simulink model "gm_hdl_model_fixed_vnl"  (R2024a)
settings: Solver=FixedStepDiscrete  StartTime=0.0  StopTime=SIM_TIME  RelTol=1e-3
model workspace (MAT data in the model file):
  HDLVAXIManagerConfig : hdlverifier.internal.AXIMaster.ConfigParams (value not decoded)
undefined symbols (not defined in the file or in its folder): a, b, BUFFER_LEN, c, SAMPLING_FREQ, signal_1
libraries: hdlsllib x40, simulink x16, simulink_extras x5, dsphdlxfrm2 x2, dspsrcs4 x1
(part 3 of 3)

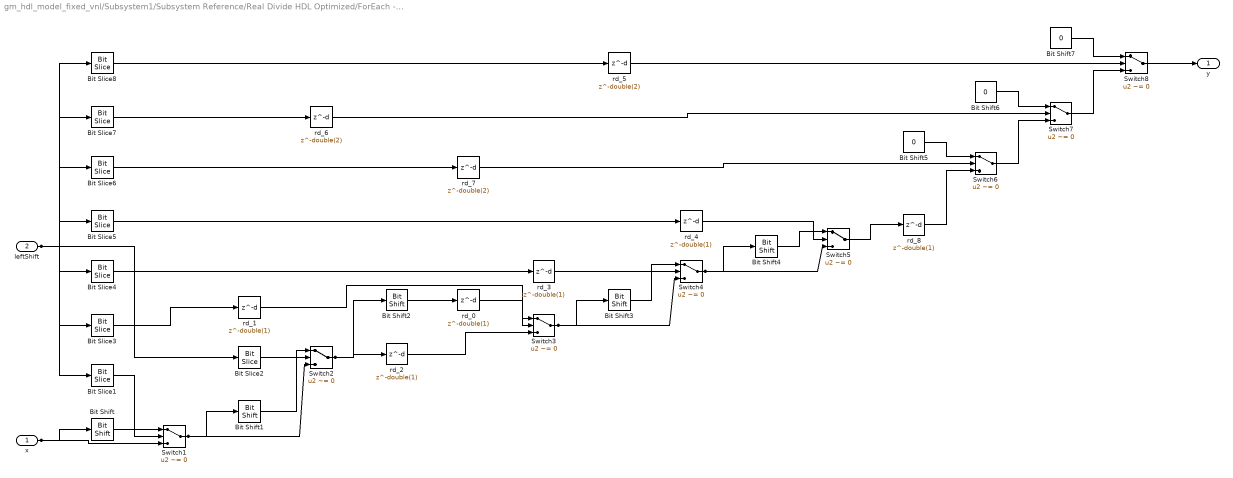
== system gm_hdl_model_fixed_vnl/Subsystem1/Subsystem Reference/Real Divide HDL Optimized/ForEach - Real Divide_instance1/Shift and cast to output type/Variable Left Shift ==
  x : Inport  OutDataTypeStr=fixdt(1, 23, 15)  SampleTime=1e-08
  leftShift : Inport  Port=2  OutDataTypeStr=int32  SampleTime=1e-08
  Bit Shift : hdlsllib/Logic and Bit Operations/Bit Shift  mode=Shift Left Logical  N=double(1)
  Bit Shift1 : hdlsllib/Logic and Bit Operations/Bit Shift  mode=Shift Left Logical  N=double(2)
  Bit Shift2 : hdlsllib/Logic and Bit Operations/Bit Shift  mode=Shift Left Logical  N=double(4)
  Bit Shift3 : hdlsllib/Logic and Bit Operations/Bit Shift  mode=Shift Left Logical  N=double(8)
  Bit Shift4 : hdlsllib/Logic and Bit Operations/Bit Shift  mode=Shift Left Logical  N=double(16)
  Bit Shift5 : Constant  Value=0  OutDataTypeStr=fixdt(1, 23, 15)  SampleTime=1e-08
  Bit Shift6 : Constant  Value=0  OutDataTypeStr=fixdt(1, 23, 15)  SampleTime=1e-08
  Bit Shift7 : Constant  Value=0  OutDataTypeStr=fixdt(1, 23, 15)  SampleTime=1e-08
  Bit Slice1 : hdlsllib/Logic and Bit Operations/Bit Slice  lidx=double(0)  ridx=double(0)
  Bit Slice2 : hdlsllib/Logic and Bit Operations/Bit Slice  lidx=double(1)  ridx=double(1)
  Bit Slice3 : hdlsllib/Logic and Bit Operations/Bit Slice  lidx=double(2)  ridx=double(2)
  Bit Slice4 : hdlsllib/Logic and Bit Operations/Bit Slice  lidx=double(3)  ridx=double(3)
  Bit Slice5 : hdlsllib/Logic and Bit Operations/Bit Slice  lidx=double(4)  ridx=double(4)
  Bit Slice6 : hdlsllib/Logic and Bit Operations/Bit Slice  lidx=double(5)  ridx=double(5)
  Bit Slice7 : hdlsllib/Logic and Bit Operations/Bit Slice  lidx=double(6)  ridx=double(6)
  Bit Slice8 : hdlsllib/Logic and Bit Operations/Bit Slice  lidx=double(7)  ridx=double(7)
  Switch{1..8} (8 alike) : Switch  Criteria=u2 ~= 0  Threshold=double(0)  OutDataTypeStr=fixdt(1, 23, 15)  SampleTime=1e-08  SaturateOnIntegerOverflow=off  InputSameDT=off
  rd_{0..4,8} (6 alike) : Delay  DelayLength=double(1)  InitialCondition=0  SampleTime=1e-08
  rd_5 : Delay  DelayLength=double(2)  InitialCondition=0  SampleTime=1e-08
  rd_6 : Delay  DelayLength=double(2)  InitialCondition=0  SampleTime=1e-08
  rd_7 : Delay  DelayLength=double(2)  InitialCondition=0  SampleTime=1e-08
  y : Outport  SampleTime=1e-08
  wires:
  rd_0/1 -> Switch3/1
  rd_1/1 -> Switch3/2
  rd_3/1 -> Switch4/2
  rd_4/1 -> Switch5/2
  rd_7/1 -> Switch6/2
  rd_6/1 -> Switch7/2
  rd_5/1 -> Switch8/2
  rd_2/1 -> Switch3/3
  rd_8/1 -> Switch6/3
  leftShift/1 -> Bit Slice8/1, Bit Slice7/1, Bit Slice6/1, Bit Slice5/1, Bit Slice4/1, Bit Slice3/1, Bit Slice2/1, Bit Slice1/1
  x/1 -> Switch1/3, Bit Shift/1
  Bit Shift/1 -> Switch1/1
  Bit Shift1/1 -> Switch2/1
  Bit Shift2/1 -> rd_0/1
  Bit Shift3/1 -> Switch4/1
  Bit Shift4/1 -> Switch5/1
  Bit Shift5/1 -> Switch6/1
  Bit Shift6/1 -> Switch7/1
  Bit Shift7/1 -> Switch8/1
  Bit Slice1/1 -> Switch1/2
  Bit Slice2/1 -> Switch2/2
  Bit Slice3/1 -> rd_1/1
  Bit Slice4/1 -> rd_3/1
  Bit Slice5/1 -> rd_4/1
  Bit Slice6/1 -> rd_7/1
  Bit Slice7/1 -> rd_6/1
  Bit Slice8/1 -> rd_5/1
  Switch1/1 -> Switch2/3, Bit Shift1/1
  Switch2/1 -> Bit Shift2/1, rd_2/1
  Switch3/1 -> Switch4/3, Bit Shift3/1
  Switch4/1 -> Switch5/3, Bit Shift4/1
  Switch5/1 -> rd_8/1
  Switch6/1 -> Switch7/3
  Switch7/1 -> Switch8/3
  Switch8/1 -> y/1

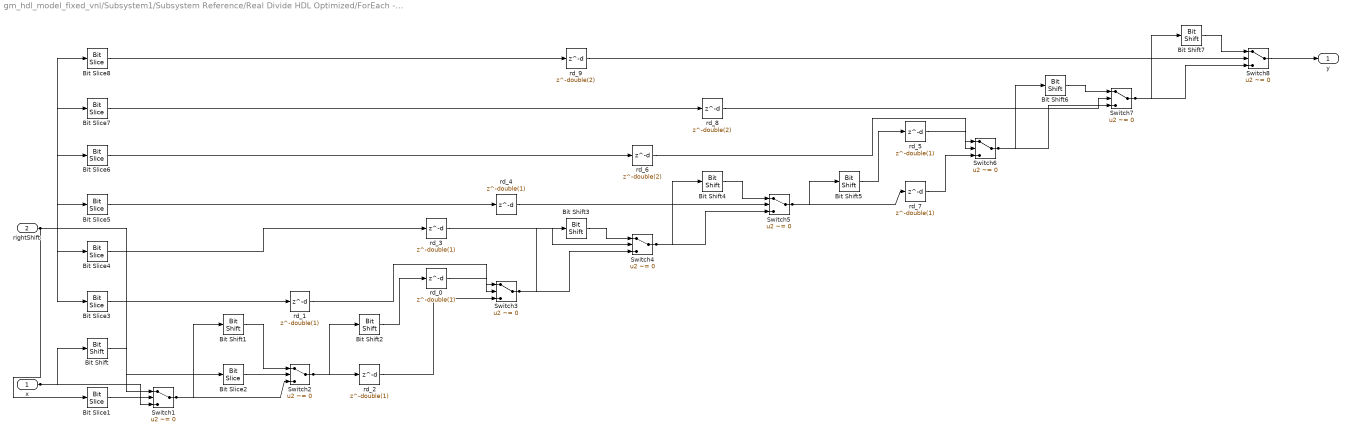
== system gm_hdl_model_fixed_vnl/Subsystem1/Subsystem Reference/Real Divide HDL Optimized/ForEach - Real Divide_instance1/Shift and cast to output type/Variable Right Shift ==
  x : Inport  OutDataTypeStr=fixdt(1, 23, 15)  SampleTime=1e-08
  rightShift : Inport  Port=2  OutDataTypeStr=int32  SampleTime=1e-08
  Bit Shift : hdlsllib/Logic and Bit Operations/Bit Shift  mode=Shift Right Arithmetic  N=double(1)
  Bit Shift1 : hdlsllib/Logic and Bit Operations/Bit Shift  mode=Shift Right Arithmetic  N=double(2)
  Bit Shift2 : hdlsllib/Logic and Bit Operations/Bit Shift  mode=Shift Right Arithmetic  N=double(4)
  Bit Shift3 : hdlsllib/Logic and Bit Operations/Bit Shift  mode=Shift Right Arithmetic  N=double(8)
  Bit Shift4 : hdlsllib/Logic and Bit Operations/Bit Shift  mode=Shift Right Arithmetic  N=double(16)
  Bit Shift5 : hdlsllib/Logic and Bit Operations/Bit Shift  mode=Shift Right Arithmetic  N=double(22)
  Bit Shift6 : hdlsllib/Logic and Bit Operations/Bit Shift  mode=Shift Right Arithmetic  N=double(22)
  Bit Shift7 : hdlsllib/Logic and Bit Operations/Bit Shift  mode=Shift Right Arithmetic  N=double(22)
  Bit Slice1 : hdlsllib/Logic and Bit Operations/Bit Slice  lidx=double(0)  ridx=double(0)
  Bit Slice2 : hdlsllib/Logic and Bit Operations/Bit Slice  lidx=double(1)  ridx=double(1)
  Bit Slice3 : hdlsllib/Logic and Bit Operations/Bit Slice  lidx=double(2)  ridx=double(2)
  Bit Slice4 : hdlsllib/Logic and Bit Operations/Bit Slice  lidx=double(3)  ridx=double(3)
  Bit Slice5 : hdlsllib/Logic and Bit Operations/Bit Slice  lidx=double(4)  ridx=double(4)
  Bit Slice6 : hdlsllib/Logic and Bit Operations/Bit Slice  lidx=double(5)  ridx=double(5)
  Bit Slice7 : hdlsllib/Logic and Bit Operations/Bit Slice  lidx=double(6)  ridx=double(6)
  Bit Slice8 : hdlsllib/Logic and Bit Operations/Bit Slice  lidx=double(7)  ridx=double(7)
  Switch{1..8} (8 alike) : Switch  Criteria=u2 ~= 0  Threshold=double(0)  OutDataTypeStr=fixdt(1, 23, 15)  SampleTime=1e-08  SaturateOnIntegerOverflow=off  InputSameDT=off
  rd_{0..5,7} (7 alike) : Delay  DelayLength=double(1)  InitialCondition=0  SampleTime=1e-08
  rd_6 : Delay  DelayLength=double(2)  InitialCondition=0  SampleTime=1e-08
  rd_8 : Delay  DelayLength=double(2)  InitialCondition=0  SampleTime=1e-08
  rd_9 : Delay  DelayLength=double(2)  InitialCondition=0  SampleTime=1e-08
  y : Outport  SampleTime=1e-08
  wires:
  rd_0/1 -> Switch3/1
  rd_5/1 -> Switch6/1
  rd_1/1 -> Switch3/2
  rd_3/1 -> Switch4/2
  rd_4/1 -> Switch5/2
  rd_6/1 -> Switch6/2
  rd_8/1 -> Switch7/2
  rd_9/1 -> Switch8/2
  rd_2/1 -> Switch3/3
  rd_7/1 -> Switch6/3
  rightShift/1 -> Bit Slice8/1, Bit Slice7/1, Bit Slice6/1, Bit Slice5/1, Bit Slice4/1, Bit Slice3/1, Bit Slice2/1, Bit Slice1/1
  x/1 -> Switch1/3, Bit Shift/1
  Bit Shift/1 -> Switch1/1
  Bit Shift1/1 -> Switch2/1
  Bit Shift2/1 -> rd_0/1
  Bit Shift3/1 -> Switch4/1
  Bit Shift4/1 -> Switch5/1
  Bit Shift5/1 -> rd_5/1
  Bit Shift6/1 -> Switch7/1
  Bit Shift7/1 -> Switch8/1
  Bit Slice1/1 -> Switch1/2
  Bit Slice2/1 -> Switch2/2
  Bit Slice3/1 -> rd_1/1
  Bit Slice4/1 -> rd_3/1
  Bit Slice5/1 -> rd_4/1
  Bit Slice6/1 -> rd_6/1
  Bit Slice7/1 -> rd_8/1
  Bit Slice8/1 -> rd_9/1
  Switch1/1 -> Switch2/3, Bit Shift1/1
  Switch2/1 -> Bit Shift2/1, rd_2/1
  Switch3/1 -> Switch4/3, Bit Shift3/1
  Switch4/1 -> Switch5/3, Bit Shift4/1
  Switch5/1 -> Bit Shift5/1, rd_7/1
  Switch6/1 -> Switch7/3, Bit Shift6/1
  Switch7/1 -> Switch8/3, Bit Shift7/1
  Switch8/1 -> y/1

== system gm_hdl_model_fixed_vnl/Subsystem1/myRMS/CORDIC Square Root HDL Optimized/Synchronous Subsystem/cordicSquareRootHDL/embmathops_c2_s84XJG1CWMolALoedlonStG_cordicSquareRootHDL_controlled ==
  in0 : Inport  OutDataTypeStr=fixdt(0, 16, 7)  SampleTime=1e-08
  in1 : Inport  Port=2  OutDataTypeStr=boolean  SampleTime=1e-08
  in2 : Inport  Port=3  OutDataTypeStr=boolean  SampleTime=1e-08
  stateControl : EnablePort  OutDataTypeStr=boolean
  embmathops_c2_s84XJG1CWMolALoedlonStG_cordicSquareRootHDL : MATLAB Function  TreatAsAtomicUnit=on
      settings: LibrarySourceBlock=embmathops/CORDIC Square Root HDL Optimized/Synchronous Subsystem/cordicSquareRootHDL
  out0 : Outport  OutDataTypeStr=fixdt(1, 16, 14)  SampleTime=1e-08  InitialOutput=0
  out1 : Outport  Port=2  OutDataTypeStr=int32  SampleTime=1e-08  InitialOutput=0
  out2 : Outport  Port=3  OutDataTypeStr=boolean  SampleTime=1e-08  InitialOutput=0
  out3 : Outport  Port=4  OutDataTypeStr=boolean  SampleTime=1e-08  InitialOutput=0
  wires:
  in2/1 -> embmathops_c2_s84XJG1CWMolALoedlonStG_cordicSquareRootHDL/3(restart)
  in1/1 -> embmathops_c2_s84XJG1CWMolALoedlonStG_cordicSquareRootHDL/2(validIn)
  in0/1 -> embmathops_c2_s84XJG1CWMolALoedlonStG_cordicSquareRootHDL/1(u)
  embmathops_c2_s84XJG1CWMolALoedlonStG_cordicSquareRootHDL/4(validOut) -> out3/1
  embmathops_c2_s84XJG1CWMolALoedlonStG_cordicSquareRootHDL/3(isZero) -> out2/1
  embmathops_c2_s84XJG1CWMolALoedlonStG_cordicSquareRootHDL/2(eOut) -> out1/1
  embmathops_c2_s84XJG1CWMolALoedlonStG_cordicSquareRootHDL/1(dataOut) -> out0/1

== system gm_hdl_model_fixed_vnl/Subsystem1/Subsystem Reference/Absolute of Complex/CORDIC Square Root HDL Optimized1/Synchronous Subsystem/cordicSquareRootHDL/embmathops_c2_srwrzER3uCGRdPfDbow0ID_cordicSquareRootHDL_controlled ==
  in0 : Inport  OutDataTypeStr=fixdt(1, 24, 22)  SampleTime=1e-08
  in1 : Inport  Port=2  OutDataTypeStr=boolean  SampleTime=1e-08
  in2 : Inport  Port=3  OutDataTypeStr=boolean  SampleTime=1e-08
  stateControl : EnablePort  OutDataTypeStr=boolean
  embmathops_c2_srwrzER3uCGRdPfDbow0ID_cordicSquareRootHDL : MATLAB Function  TreatAsAtomicUnit=on
      settings: LibrarySourceBlock=embmathops/CORDIC Square Root HDL Optimized/Synchronous Subsystem/cordicSquareRootHDL
  out0 : Outport  OutDataTypeStr=fixdt(1, 24, 22)  SampleTime=1e-08  InitialOutput=0
  out1 : Outport  Port=2  OutDataTypeStr=int32  SampleTime=1e-08  InitialOutput=0
  out2 : Outport  Port=3  OutDataTypeStr=boolean  SampleTime=1e-08  InitialOutput=0
  out3 : Outport  Port=4  OutDataTypeStr=boolean  SampleTime=1e-08  InitialOutput=0
  wires:
  in2/1 -> embmathops_c2_srwrzER3uCGRdPfDbow0ID_cordicSquareRootHDL/3(restart)
  in1/1 -> embmathops_c2_srwrzER3uCGRdPfDbow0ID_cordicSquareRootHDL/2(validIn)
  in0/1 -> embmathops_c2_srwrzER3uCGRdPfDbow0ID_cordicSquareRootHDL/1(u)
  embmathops_c2_srwrzER3uCGRdPfDbow0ID_cordicSquareRootHDL/4(validOut) -> out3/1
  embmathops_c2_srwrzER3uCGRdPfDbow0ID_cordicSquareRootHDL/3(isZero) -> out2/1
  embmathops_c2_srwrzER3uCGRdPfDbow0ID_cordicSquareRootHDL/2(eOut) -> out1/1
  embmathops_c2_srwrzER3uCGRdPfDbow0ID_cordicSquareRootHDL/1(dataOut) -> out0/1

== system gm_hdl_model_fixed_vnl/Subsystem1/Subsystem Reference/Real Divide HDL Optimized/ForEach - Real Divide_instance1/Divide real numerator by denominator/normalizedCORDICDivide/embreciprocals_c21_normalizedCORDICDivide_controlled ==
  in0 : Inport  OutDataTypeStr=fixdt(1, 17, 15)  SampleTime=1e-08
  in1 : Inport  Port=2  OutDataTypeStr=fixdt(1, 17, 15)  SampleTime=1e-08
  in2 : Inport  Port=3  OutDataTypeStr=fixdt(1, 33, 0)  SampleTime=1e-08
  in3 : Inport  Port=4  OutDataTypeStr=int32  SampleTime=1e-08
  in4 : Inport  Port=5  OutDataTypeStr=boolean  SampleTime=1e-08
  in5 : Inport  Port=6  OutDataTypeStr=boolean  SampleTime=1e-08
  in6 : Inport  Port=7  OutDataTypeStr=boolean  SampleTime=1e-08
  stateControl : EnablePort  OutDataTypeStr=boolean
  embreciprocals_c21_normalizedCORDICDivide : MATLAB Function  TreatAsAtomicUnit=on
      settings: LibrarySourceBlock=embreciprocals/Divide real numerator by denominator/normalizedCORDICDivide
  out0 : Outport  OutDataTypeStr=fixdt(1, 17, 15)  SampleTime=1e-08  InitialOutput=0
  out1 : Outport  Port=2  OutDataTypeStr=fixdt(1, 34, 0)  SampleTime=1e-08  InitialOutput=0
  out2 : Outport  Port=3  OutDataTypeStr=boolean  SampleTime=1e-08  InitialOutput=0
  out3 : Outport  Port=4  OutDataTypeStr=boolean  SampleTime=1e-08  InitialOutput=0
  wires:
  in6/1 -> embreciprocals_c21_normalizedCORDICDivide/7(validIn)
  in5/1 -> embreciprocals_c21_normalizedCORDICDivide/6(isDenNegative)
  in4/1 -> embreciprocals_c21_normalizedCORDICDivide/5(isNumNegative)
  in3/1 -> embreciprocals_c21_normalizedCORDICDivide/4(tDen)
  in2/1 -> embreciprocals_c21_normalizedCORDICDivide/3(tNum)
  in1/1 -> embreciprocals_c21_normalizedCORDICDivide/2(den)
  in0/1 -> embreciprocals_c21_normalizedCORDICDivide/1(num)
  embreciprocals_c21_normalizedCORDICDivide/4(validOut) -> out3/1
  embreciprocals_c21_normalizedCORDICDivide/3(isDenZeroOut) -> out2/1
  embreciprocals_c21_normalizedCORDICDivide/2(t) -> out1/1
  embreciprocals_c21_normalizedCORDICDivide/1(y) -> out0/1

== system gm_hdl_model_fixed_vnl/Subsystem1/Subsystem Reference/Real Divide HDL Optimized/ForEach - Real Divide_instance1/Normalize denominator/positiveRealNormalizer/embreciprocals_c3_positiveRealNormalizer_controlled ==
  in0 : Inport  OutDataTypeStr=fixdt(1, 17, 14)  SampleTime=1e-08
  in1 : Inport  Port=2  OutDataTypeStr=boolean  SampleTime=1e-08
  stateControl : EnablePort  OutDataTypeStr=boolean
  embreciprocals_c3_positiveRealNormalizer : MATLAB Function  TreatAsAtomicUnit=on
      settings: LibrarySourceBlock=embreciprocals/Real Normalizer HDL Optimized/positiveRealNormalizer
  out0 : Outport  OutDataTypeStr=fixdt(1, 17, 15)  SampleTime=1e-08  InitialOutput=0
  out1 : Outport  Port=2  OutDataTypeStr=int32  SampleTime=1e-08  InitialOutput=0
  out2 : Outport  Port=3  OutDataTypeStr=boolean  SampleTime=1e-08  InitialOutput=0
  out3 : Outport  Port=4  OutDataTypeStr=boolean  SampleTime=1e-08  InitialOutput=0
  wires:
  in1/1 -> embreciprocals_c3_positiveRealNormalizer/2(validIn)
  in0/1 -> embreciprocals_c3_positiveRealNormalizer/1(u)
  embreciprocals_c3_positiveRealNormalizer/4(validOut) -> out3/1
  embreciprocals_c3_positiveRealNormalizer/3(isNegative) -> out2/1
  embreciprocals_c3_positiveRealNormalizer/2(e) -> out1/1
  embreciprocals_c3_positiveRealNormalizer/1(x) -> out0/1

== system gm_hdl_model_fixed_vnl/Subsystem1/Subsystem Reference/Real Divide HDL Optimized/ForEach - Real Divide_instance1/Normalize numerator/positiveRealNormalizer/embreciprocals_c3_positiveRealNormalizer_controlled ==
  in0 : Inport  OutDataTypeStr=fixdt(1, 17, 14)  SampleTime=1e-08
  in1 : Inport  Port=2  OutDataTypeStr=boolean  SampleTime=1e-08
  stateControl : EnablePort  OutDataTypeStr=boolean
  embreciprocals_c3_positiveRealNormalizer : MATLAB Function  TreatAsAtomicUnit=on
      settings: LibrarySourceBlock=embreciprocals/Real Normalizer HDL Optimized/positiveRealNormalizer
  out0 : Outport  OutDataTypeStr=fixdt(1, 17, 15)  SampleTime=1e-08  InitialOutput=0
  out1 : Outport  Port=2  OutDataTypeStr=int32  SampleTime=1e-08  InitialOutput=0
  out2 : Outport  Port=3  OutDataTypeStr=boolean  SampleTime=1e-08  InitialOutput=0
  out3 : Outport  Port=4  OutDataTypeStr=boolean  SampleTime=1e-08  InitialOutput=0
  wires:
  in1/1 -> embreciprocals_c3_positiveRealNormalizer/2(validIn)
  in0/1 -> embreciprocals_c3_positiveRealNormalizer/1(u)
  embreciprocals_c3_positiveRealNormalizer/4(validOut) -> out3/1
  embreciprocals_c3_positiveRealNormalizer/3(isNegative) -> out2/1
  embreciprocals_c3_positiveRealNormalizer/2(e) -> out1/1
  embreciprocals_c3_positiveRealNormalizer/1(x) -> out0/1

== matlab function gm_hdl_model_fixed_vnl/Subsystem1/Subsystem Reference/Real Divide HDL Optimized/ForEach - Real Divide_instance1/Normalize numerator/positiveRealNormalizer/embreciprocals_c3_positiveRealNormalizer_controlled/embreciprocals_c3_positiveRealNormalizer ==
  settings: fimath=hdlfimath
  data: u input; x output; validIn input; e output; isNegative output; validOut output
function [x, e, isNegative, validOut] = realNormalizer(u, validIn)
    %realNormalizer Normalize real values.
    % Given real scalar u ~= 0, this block produces x such that
    %    1 <= x < 2,
    % e such that
    %    x = (2^e)*|u|,
    % and isNegative = u<0.
    %
    %   When u = 0 and u is fixed-point or scaled-double, then x = 0 and
    %   e = (2^nextpow2(x.WordLength)) - x.WordLength - x.FractionLength.
    %
    %   When u = 0 and u is floating-point, then x = 0 and e = 1.
    
    %   Copyright 2019 The MathWorks, Inc.
    %#codegen
    
    % This function only works on scalars.
    % Only operate on the real part
    fixed.internal.reciprocal.validateNormalizerInputs(u, validIn);
    % Normalize in unsigned type.
    [x_normalized, n_normalized, isNegative, validOut] = normalize(real(u), validIn);
    % Cast the output to signed if the input was signed.
    x = fixed.internal.reciprocal.castToInputSignedness(x_normalized,u);
    % Convert the normalized shift value based on the data type of the
    % input U so that the output of the normalizer X is in real-world
    % scale and X = (2^N)*U.
    e = fi(int32(0));
    e(:) = fixed.internal.reciprocal.normalizedShiftToRealWorldValueShift(n_normalized,u);
end

function [x_normalized, e_normalized, isNegative, validOut] = normalize(u, validIn)
    [u, isNegative] = fixed.reciprocal.pipelined.makeRealScalarPositive(u);
    if isfi(u) && isfixed(u)
        % Normalize fixed-point values
        [x_normalized, e_normalized, isNegative, validOut] = normalizeFixedpoint(u, isNegative, validIn);
    else
        % Normalize floating-point or scaled-double
        [x_normalized, e_normalized, validOut] = fixed.internal.reciprocal.normalizePositiveFloatOrScaledDouble(u, validIn);
    end
end

function [u_normalized, e_normalized, isNegativeOut, validOut] = normalizeFixedpoint(u, isNegative, validIn)
    % Normalize fixed-point values.
    persistent validReg
    persistent tReg
    persistent xReg
    persistent isNegativeReg
    % For fixed-point types, the normalization uses a binary search of
    % length log2 of the word length of the input.
    number_of_stages = coder.const(nextpow2(u.WordLength));
    
    if isempty(validReg)
        validReg = false(number_of_stages+1,1);
        tReg = zeros(number_of_stages+1,1,'like',fi(0,0,max(number_of_stages,1),0));
        xReg = zeros(number_of_stages+1,1,'like',fi([],0,u.WordLength,0));
        isNegativeReg = false(number_of_stages+1,1);
    end
    
    [u_normalized, e_normalized,validOut,...
        validReg, tReg,xReg...  % Persistent
        ] = fixed.internal.reciprocal.normalizePositiveFixedPoint(u, validIn, number_of_stages, ...
        validReg, tReg,xReg...  % Persistent
        );
    % Assign outputs from states
    isNegativeOut = isNegativeReg(end);
    
    % Update isNegative states
    coder.unroll;
    for k = number_of_stages:-1:1
        isNegativeReg(k+1) = isNegativeReg(k);
    end
    isNegativeReg(1) = isNegative;
end

== matlab function gm_hdl_model_fixed_vnl/Subsystem1/Subsystem Reference/Real Divide HDL Optimized/Reshape to original size/embreciprocals_c11_Reshape_to_original_size ==
  data: y input; u input; z output
function z = reshape_to_original_size(y,u)
    z = reshape(y,size(u));
end

== matlab function gm_hdl_model_fixed_vnl/Subsystem1/Subsystem Reference/Real Divide HDL Optimized/ForEach - Real Divide_instance1/Normalize denominator/positiveRealNormalizer/embreciprocals_c3_positiveRealNormalizer_controlled/embreciprocals_c3_positiveRealNormalizer ==
  settings: fimath=hdlfimath
  data: u input; x output; validIn input; e output; isNegative output; validOut output
function [x, e, isNegative, validOut] = realNormalizer(u, validIn)
    %realNormalizer Normalize real values.
    % Given real scalar u ~= 0, this block produces x such that
    %    1 <= x < 2,
    % e such that
    %    x = (2^e)*|u|,
    % and isNegative = u<0.
    %
    %   When u = 0 and u is fixed-point or scaled-double, then x = 0 and
    %   e = (2^nextpow2(x.WordLength)) - x.WordLength - x.FractionLength.
    %
    %   When u = 0 and u is floating-point, then x = 0 and e = 1.
    
    %   Copyright 2019 The MathWorks, Inc.
    %#codegen
    
    % This function only works on scalars.
    % Only operate on the real part
    fixed.internal.reciprocal.validateNormalizerInputs(u, validIn);
    % Normalize in unsigned type.
    [x_normalized, n_normalized, isNegative, validOut] = normalize(real(u), validIn);
    % Cast the output to signed if the input was signed.
    x = fixed.internal.reciprocal.castToInputSignedness(x_normalized,u);
    % Convert the normalized shift value based on the data type of the
    % input U so that the output of the normalizer X is in real-world
    % scale and X = (2^N)*U.
    e = fi(int32(0));
    e(:) = fixed.internal.reciprocal.normalizedShiftToRealWorldValueShift(n_normalized,u);
end

function [x_normalized, e_normalized, isNegative, validOut] = normalize(u, validIn)
    [u, isNegative] = fixed.reciprocal.pipelined.makeRealScalarPositive(u);
    if isfi(u) && isfixed(u)
        % Normalize fixed-point values
        [x_normalized, e_normalized, isNegative, validOut] = normalizeFixedpoint(u, isNegative, validIn);
    else
        % Normalize floating-point or scaled-double
        [x_normalized, e_normalized, validOut] = fixed.internal.reciprocal.normalizePositiveFloatOrScaledDouble(u, validIn);
    end
end

function [u_normalized, e_normalized, isNegativeOut, validOut] = normalizeFixedpoint(u, isNegative, validIn)
    % Normalize fixed-point values.
    persistent validReg
    persistent tReg
    persistent xReg
    persistent isNegativeReg
    % For fixed-point types, the normalization uses a binary search of
    % length log2 of the word length of the input.
    number_of_stages = coder.const(nextpow2(u.WordLength));
    
    if isempty(validReg)
        validReg = false(number_of_stages+1,1);
        tReg = zeros(number_of_stages+1,1,'like',fi(0,0,max(number_of_stages,1),0));
        xReg = zeros(number_of_stages+1,1,'like',fi([],0,u.WordLength,0));
        isNegativeReg = false(number_of_stages+1,1);
    end
    
    [u_normalized, e_normalized,validOut,...
        validReg, tReg,xReg...  % Persistent
        ] = fixed.internal.reciprocal.normalizePositiveFixedPoint(u, validIn, number_of_stages, ...
        validReg, tReg,xReg...  % Persistent
        );
    % Assign outputs from states
    isNegativeOut = isNegativeReg(end);
    
    % Update isNegative states
    coder.unroll;
    for k = number_of_stages:-1:1
        isNegativeReg(k+1) = isNegativeReg(k);
    end
    isNegativeReg(1) = isNegative;
end

== matlab function gm_hdl_model_fixed_vnl/Subsystem1/Subsystem Reference/Real Divide HDL Optimized/ForEach - Real Divide_instance1/Upcast Wordlength/slutils_c2_Upcast_Wordlength ==
  data: x input; u output; y input; v output
function [u, v] = upcastWordlength(x, y)

% Copyright 2019 The MathWorks, Inc.

%#codegen

[u, v] = fixed.internal.type.upcastWordlength(x,y);

end

== matlab function gm_hdl_model_fixed_vnl/Subsystem1/Subsystem Reference/Real Divide HDL Optimized/ForEach - Real Divide_instance1/MATLAB Function/embreciprocals_c13_MATLAB_Function ==
  settings: fimath=hdlfimath
  data: num input; num_out output; t_num input; t_num_out output
function [num_out, t_num_out] = fcn(num, t_num)

num_out = bitsra(num,1);
t_num_out = t_num - 1;

end

== matlab function gm_hdl_model_fixed_vnl/Subsystem1/myRMS/CORDIC Square Root HDL Optimized/Synchronous Subsystem/cordicSquareRootHDL/embmathops_c2_s84XJG1CWMolALoedlonStG_cordicSquareRootHDL_controlled/embmathops_c2_s84XJG1CWMolALoedlonStG_cordicSquareRootHDL ==
  settings: fimath=hdlfimath
  data: u input; dataOut output; validIn input; restart input; eOut output; isZero output; validOut output; maximumShiftValue parameter; nIterPerReg parameter; autoMaximumShiftVal parameter
function [dataOut,eOut,isZero,validOut] = cordicSquareRootHDL(u,validIn,restart,maximumShiftValue, nIterPerReg, autoMaximumShiftVal)
    % [dataOut,eOut,validOut] = cordicSquareRootHDL(u,validIn,restart,maximumShiftValue,nIterPerReg)
    % This function computes the normalized square root of input data u
    % based on CORDIC hyperbolic vectoring mode. eOut is the bit shift
    % value to be used during denormalization.
    %
    % This function first performs normalization of input u and then
    % computes square root of normalized u using CORDIC hyperbolic
    % vectoring mode.

    %   Copyright 2023 The MathWorks, Inc.

    %#codegen
    
    fixed.internal.reciprocal.validateNormalizerInputs(u, validIn);

    %% Constants
    if autoMaximumShiftVal
        N = coder.const(fixed.cordic.maximumShiftValue(u));
    else
        N = coder.const(maximumShiftValue);
    end

    Kn = coder.const(fixed.cordic.hyperbolic.inverseScaleFactor(N));
    INITOFFSET = coder.const(0.25);
    shiftSeq = coder.const(fixed.cordic.hyperbolic.shiftSequence(N));
    nCORDICIterations = coder.const(length(shiftSeq));

    %% Run CORDIC square root workflow
    uPos = fixed.cordic.linear.makeRealScalarPositiveUnsigned(u);
    if isfi(u)&&isscaledtype(u)
        coder.internal.assert(u.WordLength>N,'fixed:emblib:CORDICMaxShiftValMustBeSmallerThanWordlength');
        [dataOut, eOut, isZero, validOut] = sqrtIterFixed(uPos, validIn, restart,nIterPerReg,Kn,INITOFFSET,shiftSeq,nCORDICIterations);
    else
        [dataOut, eOut] = fixed.emblib.cordicsqrt.cordicSqrtFloat(uPos, Kn, INITOFFSET, shiftSeq, nCORDICIterations);
        validOut = validIn;
        isZero = u==0;
    end
end

function [dataOut, eOut, isZero, validOut] = sqrtIterFixed(u, validIn, restart, nIterPerReg, Kn, INITOFFSET, shiftSeq, nCORDICIterations)
        uInt = stripscaling(u);
        
        wordLength = coder.const(uInt.WordLength);
        normalizerType = numerictype(1,32,0);

        % CORDIC datatype and corresponding fimath
        CORDICprototype = fi([],1,wordLength,wordLength-2,'DataType',uInt.DataType);
        Fxy = fixed.fimathLike(CORDICprototype);
        
        % Allocate registers
        [numOfNormSteps,nNormReg,normInd,nTrailingNormSteps,trailingNormIdx,nLeadingCORDICSteps,nCORDICReg,CORDICShiftInd,nTotReg]...
            = fixed.emblib.cordicsqrt.allocateReg(wordLength,nCORDICIterations,nIterPerReg);
        
        %% Registers
        persistent xRegNorm xRegCORDIC yReg eRegNorm eRegCORDIC validReg dataOutReg eOutReg isZeroReg
        if isempty(xRegNorm)
            xRegNorm = zeros(nNormReg,1,'like',uInt);
            xRegCORDIC = setfimath(zeros(nCORDICReg,1,'like',CORDICprototype),Fxy);
            yReg = setfimath(zeros(nCORDICReg,1,'like',CORDICprototype),Fxy);
            eRegNorm = fi(zeros(nNormReg,1),0,numOfNormSteps,0);
            eRegCORDIC = fi(zeros(nCORDICReg,1),normalizerType);
            validReg = false(nTotReg+1,1);
            dataOutReg = setfimath(cast(0,'like',CORDICprototype),Fxy);
            eOutReg = fi(0,normalizerType);
            isZeroReg = false(nTotReg+1,1);
        end
        
        %% Assign outputs
        dataOut = dataOutReg;
        eOut = eOutReg;
        validOut = validReg(end);
        isZero = isZeroReg(end);
        
        %% Update registers
        [xRegNorm, xRegCORDIC, yReg, eRegNorm, eRegCORDIC, validReg, dataOutReg, eOutReg, isZeroReg]...
        = fixed.emblib.cordicsqrt.cordicSqrtFiScaledtypeUpdateReg(u, uInt, validIn, restart,... % Inputs
        xRegNorm, xRegCORDIC, yReg, eRegNorm, eRegCORDIC, validReg, dataOutReg, eOutReg, isZeroReg,... %Registers
        Kn, INITOFFSET, shiftSeq, nIterPerReg,... % Constants for algorithms
        nTotReg, nNormReg, CORDICShiftInd, normInd, nTrailingNormSteps, trailingNormIdx, nLeadingCORDICSteps); % Constants for partition algorithms
end

== matlab function gm_hdl_model_fixed_vnl/Subsystem1/BUF_MIN_MAX_AVG/MATLAB Function1/MATLAB Function1 ==
  data: input_data input; max_out output; reset input
function max_out = stream_max(input_data, reset)
    % input_data: Input data stream (e.g., 16-bit integer)
    % reset: Reset signal (active high)

    % Persistent variable to hold the current maximum value
    persistent current_max;
    
    % Initialize persistent variable if it's the first time the function is called
    if isempty(current_max)
        current_max = fi(-0.5, 1, 12, 11); % Set initial maximum to a very small value (-inf)
    end
    
    % On reset, set the maximum value back to a very small value
    if reset
        current_max = fi(-0.5, 1, 12, 11); % Set to the smallest value for fixed-point
    else
        % Update the current maximum on each clock cycle
        if input_data > current_max
            current_max = input_data;
        end
    end
    
    % Output the current maximum value
    max_out = current_max;
end

== matlab function gm_hdl_model_fixed_vnl/Subsystem1/Subsystem Reference/Real Divide HDL Optimized/y = u(1)/embreciprocals_c16_y___u_1_ ==
  data: u input; y output
function y = select_one(u)
    y = u(1);
end

== matlab function gm_hdl_model_fixed_vnl/Subsystem1/myRMS/CORDIC Square Root HDL Optimized/Bit Shift Arithmetic/embmathops_c6_st99WwhDyWfnOmuPiiKPkxE_Bit_Shift_Arithmetic ==
  settings: fimath=hdlfimath
  data: u input; y output; e input; isZero input
function y = bitShiftArithmetic(u,e,isZero)
%#codegen
if isZero
    y = cast(0,'like',u);
else
    if e<0
        y = bitsll(u,-e);
    else
        y = bitsra(u,e);
    end
end

== matlab function gm_hdl_model_fixed_vnl/Subsystem1/myRMS/CORDIC Square Root HDL Optimized/Cast to Union of Types/slutils_c1_sjX4rJHbVvOr6YSpugZXv9B_Cast_to_Union_of_Types ==
  settings: fimath=hdlfimath
  data: Xref input; Cout output; Cin input
function Cout = castToUnionType(Xref,Cin)
    %castToUnionType Cast second input to union of the two types
    if (isfloat(Xref) && isfloat(Cin)) || (isFixed(Xref) && isFixed(Cin))
        T = fixed.internal.type.unionPrototype(Cin,Xref,...
        'RoundingMethod','Floor',...
        'OverflowAction','Wrap');
        Cout = cast(Cin,'like',T);
    else
        coder.internal.assert(false,'fixed:emblib:InputOutputMustBeAllFixedOrFloat');
    end
end

function t = isFixed(x)
    t = (isfi(x) || isa(x,'embedded.numerictype')) && isscalingbinarypoint(x) ...
        || isinteger(x);
end

== matlab function gm_hdl_model_fixed_vnl/Subsystem1/Subsystem Reference/Real Divide HDL Optimized/Verify divide sizes/embreciprocals_c19_Verify_divide_sizes ==
  data: denominator input; den output; numerator input; num output
function [den,num] = verify_size(denominator,numerator)
   % Verify that the dimensions of the input arrays match, and then reshape
   % them.
   coder.internal.assert(numel(denominator)==numel(numerator),...
       'fixed:emblib:DivideDimensionsShouldMatch',...
       'Real Divide HDL Optimized');
   num = reshape(numerator,1,numel(numerator));
   den = reshape(denominator,1,numel(denominator));
end

== matlab function gm_hdl_model_fixed_vnl/Subsystem1/Subsystem Reference/Real Divide HDL Optimized/ForEach - Real Divide_instance1/Divide real numerator by denominator/normalizedCORDICDivide/embreciprocals_c21_normalizedCORDICDivide_controlled/embreciprocals_c21_normalizedCORDICDivide ==
  settings: fimath=hdlfimath
  data: num input; den input; tNum input; tDen input; isNumNegative input; isDenNegative input; y output; t output; isDenZeroOut output; validIn input; validOut output
function [y, t, isDenZeroOut, validOut] = normalizedCORDICDivide(num, den, tNum, tDen, isNumNegative, isDenNegative, validIn)
    %   Copyright 2020 The MathWorks, Inc.
    %#codegen
    fixed.internal.reciprocal.validateReciprocalInputs(num, validIn);
    if isfi(num) && isscaledtype(num)
        isDenZero = den==0;
        isNumZero = num==0;
        % CORDIC divide for fixed-point and scaled-double types
        [y,t,isNegative,isNumZeroOut, isDenZeroOut,validOut] = fixedpointDivide(den,num,tDen-tNum,isNumNegative ~= isDenNegative, isNumZero, isDenZero,validIn);
    else
        % y = num/den for builtin types.
        y = num./den;
        t = tDen - tNum;
        isNegative = isNumNegative ~= isDenNegative;
        validOut = validIn;
        isDenZeroOut = false;
        isNumZeroOut = false;
    end
    if isNumZeroOut
        % Negate with saturate so the most negative value doesn't overflow.
        F = fimath('OverflowAction', 'Saturate');
        y(:) = setfimath(0,F);
    else
        if isNegative
            % Negate with saturate so the most negative value doesn't overflow.
            F = fimath('OverflowAction', 'Saturate');
            y(:) = -setfimath(y,F);
        end
    end
end

function [division, t, isNegativeOut, isNumZeroOut, isDenZeroOut, validOut] = fixedpointDivide(x,y,t_in,isNegative,isNumZero,isDenZero,validIn)
    T = fixed.cordic.linear.positiveReciprocalTypes(x);
    maximumShiftValue = coder.const(fixed.cordic.maximumShiftValue(T.data));
    % Register variables for the CORDIC Divide Kernel
    persistent xReg yReg zReg validReg tReg isNegativeReg isNumZeroReg isDenZeroReg
    if isempty(xReg)
        xReg = zeros(maximumShiftValue+2,1,'like',T.data);
        yReg = zeros(maximumShiftValue+2,1,'like',T.data);
        zReg = zeros(maximumShiftValue+2,1,'like',T.data);
        validReg = zeros(maximumShiftValue+2,1,'like',validIn);
        tReg = zeros(maximumShiftValue+2,1,'like',t_in);
        isNegativeReg = false(maximumShiftValue+2,1);
        isDenZeroReg = false(maximumShiftValue+2,1);
        isNumZeroReg = false(maximumShiftValue+2,1);
    end
    % CORDIC Divide Kernel
    [division,t,validOut,...
        xReg,yReg,zReg,validReg,tReg... % Persistent variables
        ] = fixed.internal.reciprocal.cordicDivideKernel(x,y,t_in,validIn,...
        xReg,yReg,zReg,validReg,tReg... % Persistent variables
        );
    
    % Assign outputs from states
    isNegativeOut = isNegativeReg(end);
    isNumZeroOut = isNumZeroReg(end);
    isDenZeroOut = isDenZeroReg(end);
    % Update isNegative states
    coder.unroll
    for k = maximumShiftValue+1:-1:1
        isNegativeReg(k+1) = isNegativeReg(k);
        isNumZeroReg(k+1) = isNumZeroReg(k);
        isDenZeroReg(k+1) = isDenZeroReg(k);
    end
    isNegativeReg(1) = isNegative;
    isNumZeroReg(1) = isNumZero;
    isDenZeroReg(1) = isDenZero;
end

== matlab function gm_hdl_model_fixed_vnl/Subsystem1/BUF_MIN_MAX_AVG/MATLAB Function/MATLAB Function ==
  data: input_data input; min_out output; reset input
function min_out = stream_min(input_data, reset)
    % input_data: Input data stream (e.g., 16-bit integer)
    % reset: Reset signal (active high)
    % clk: Clock signal for sequential logic

    % Persistent variable to hold the current minimum value
    persistent current_min;
    
    % Initialize persistent variable if it's the first time the function is called
    if isempty(current_min)
        current_min = fi(0.5, 1, 12, 11); % Set initial minimum to infinity
    end
    
    % On reset, set the minimum value back to infinity
    if reset
        current_min = fi(0.5, 1, 12, 11);
    else
        % Update the current minimum on each clock cycle
        if input_data < current_min
            current_min = input_data;
        end
    end
    
    % Output the current minimum value
    min_out = current_min;
end

== matlab function gm_hdl_model_fixed_vnl/Subsystem1/Subsystem Reference/Absolute of Complex/CORDIC Square Root HDL Optimized1/Synchronous Subsystem/cordicSquareRootHDL/embmathops_c2_srwrzER3uCGRdPfDbow0ID_cordicSquareRootHDL_controlled/embmathops_c2_srwrzER3uCGRdPfDbow0ID_cordicSquareRootHDL ==
  settings: fimath=hdlfimath
  data: u input; dataOut output; validIn input; restart input; eOut output; isZero output; validOut output; maximumShiftValue parameter; nIterPerReg parameter; autoMaximumShiftVal parameter
function [dataOut,eOut,isZero,validOut] = cordicSquareRootHDL(u,validIn,restart,maximumShiftValue, nIterPerReg, autoMaximumShiftVal)
    % [dataOut,eOut,validOut] = cordicSquareRootHDL(u,validIn,restart,maximumShiftValue,nIterPerReg)
    % This function computes the normalized square root of input data u
    % based on CORDIC hyperbolic vectoring mode. eOut is the bit shift
    % value to be used during denormalization.
    %
    % This function first performs normalization of input u and then
    % computes square root of normalized u using CORDIC hyperbolic
    % vectoring mode.

    %   Copyright 2023 The MathWorks, Inc.

    %#codegen
    
    fixed.internal.reciprocal.validateNormalizerInputs(u, validIn);

    %% Constants
    if autoMaximumShiftVal
        N = coder.const(fixed.cordic.maximumShiftValue(u));
    else
        N = coder.const(maximumShiftValue);
    end

    Kn = coder.const(fixed.cordic.hyperbolic.inverseScaleFactor(N));
    INITOFFSET = coder.const(0.25);
    shiftSeq = coder.const(fixed.cordic.hyperbolic.shiftSequence(N));
    nCORDICIterations = coder.const(length(shiftSeq));

    %% Run CORDIC square root workflow
    uPos = fixed.cordic.linear.makeRealScalarPositiveUnsigned(u);
    if isfi(u)&&isscaledtype(u)
        coder.internal.assert(u.WordLength>N,'fixed:emblib:CORDICMaxShiftValMustBeSmallerThanWordlength');
        [dataOut, eOut, isZero, validOut] = sqrtIterFixed(uPos, validIn, restart,nIterPerReg,Kn,INITOFFSET,shiftSeq,nCORDICIterations);
    else
        [dataOut, eOut] = fixed.emblib.cordicsqrt.cordicSqrtFloat(uPos, Kn, INITOFFSET, shiftSeq, nCORDICIterations);
        validOut = validIn;
        isZero = u==0;
    end
end

function [dataOut, eOut, isZero, validOut] = sqrtIterFixed(u, validIn, restart, nIterPerReg, Kn, INITOFFSET, shiftSeq, nCORDICIterations)
        uInt = stripscaling(u);
        
        wordLength = coder.const(uInt.WordLength);
        normalizerType = numerictype(1,32,0);

        % CORDIC datatype and corresponding fimath
        CORDICprototype = fi([],1,wordLength,wordLength-2,'DataType',uInt.DataType);
        Fxy = fixed.fimathLike(CORDICprototype);
        
        % Allocate registers
        [numOfNormSteps,nNormReg,normInd,nTrailingNormSteps,trailingNormIdx,nLeadingCORDICSteps,nCORDICReg,CORDICShiftInd,nTotReg]...
            = fixed.emblib.cordicsqrt.allocateReg(wordLength,nCORDICIterations,nIterPerReg);
        
        %% Registers
        persistent xRegNorm xRegCORDIC yReg eRegNorm eRegCORDIC validReg dataOutReg eOutReg isZeroReg
        if isempty(xRegNorm)
            xRegNorm = zeros(nNormReg,1,'like',uInt);
            xRegCORDIC = setfimath(zeros(nCORDICReg,1,'like',CORDICprototype),Fxy);
            yReg = setfimath(zeros(nCORDICReg,1,'like',CORDICprototype),Fxy);
            eRegNorm = fi(zeros(nNormReg,1),0,numOfNormSteps,0);
            eRegCORDIC = fi(zeros(nCORDICReg,1),normalizerType);
            validReg = false(nTotReg+1,1);
            dataOutReg = setfimath(cast(0,'like',CORDICprototype),Fxy);
            eOutReg = fi(0,normalizerType);
            isZeroReg = false(nTotReg+1,1);
        end
        
        %% Assign outputs
        dataOut = dataOutReg;
        eOut = eOutReg;
        validOut = validReg(end);
        isZero = isZeroReg(end);
        
        %% Update registers
        [xRegNorm, xRegCORDIC, yReg, eRegNorm, eRegCORDIC, validReg, dataOutReg, eOutReg, isZeroReg]...
        = fixed.emblib.cordicsqrt.cordicSqrtFiScaledtypeUpdateReg(u, uInt, validIn, restart,... % Inputs
        xRegNorm, xRegCORDIC, yReg, eRegNorm, eRegCORDIC, validReg, dataOutReg, eOutReg, isZeroReg,... %Registers
        Kn, INITOFFSET, shiftSeq, nIterPerReg,... % Constants for algorithms
        nTotReg, nNormReg, CORDICShiftInd, normInd, nTrailingNormSteps, trailingNormIdx, nLeadingCORDICSteps); % Constants for partition algorithms
end

== matlab function gm_hdl_model_fixed_vnl/Subsystem1/Subsystem Reference/Absolute of Complex/CORDIC Square Root HDL Optimized1/Cast to Union of Types/slutils_c1_sJq36p6JfwxqYYDPRgb8M6G_Cast_to_Union_of_Types ==
  settings: fimath=hdlfimath
  data: Xref input; Cout output; Cin input
function Cout = castToUnionType(Xref,Cin)
    %castToUnionType Cast second input to union of the two types
    if (isfloat(Xref) && isfloat(Cin)) || (isFixed(Xref) && isFixed(Cin))
        T = fixed.internal.type.unionPrototype(Cin,Xref,...
        'RoundingMethod','Floor',...
        'OverflowAction','Wrap');
        Cout = cast(Cin,'like',T);
    else
        coder.internal.assert(false,'fixed:emblib:InputOutputMustBeAllFixedOrFloat');
    end
end

function t = isFixed(x)
    t = (isfi(x) || isa(x,'embedded.numerictype')) && isscalingbinarypoint(x) ...
        || isinteger(x);
end

== matlab function gm_hdl_model_fixed_vnl/Subsystem1/Subsystem Reference/CORDIC Square Root HDL Optimized/Synchronous Subsystem/cordicSquareRootHDL/embmathops_c2_skVmLPFzLIK224pVNfQB1qF_cordicSquareRootHDL_controlled/embmathops_c2_skVmLPFzLIK224pVNfQB1qF_cordicSquareRootHDL ==
  settings: fimath=hdlfimath
  data: u input; dataOut output; validIn input; restart input; eOut output; isZero output; validOut output; maximumShiftValue parameter; nIterPerReg parameter; autoMaximumShiftVal parameter
function [dataOut,eOut,isZero,validOut] = cordicSquareRootHDL(u,validIn,restart,maximumShiftValue, nIterPerReg, autoMaximumShiftVal)
    % [dataOut,eOut,validOut] = cordicSquareRootHDL(u,validIn,restart,maximumShiftValue,nIterPerReg)
    % This function computes the normalized square root of input data u
    % based on CORDIC hyperbolic vectoring mode. eOut is the bit shift
    % value to be used during denormalization.
    %
    % This function first performs normalization of input u and then
    % computes square root of normalized u using CORDIC hyperbolic
    % vectoring mode.

    %   Copyright 2023 The MathWorks, Inc.

    %#codegen
    
    fixed.internal.reciprocal.validateNormalizerInputs(u, validIn);

    %% Constants
    if autoMaximumShiftVal
        N = coder.const(fixed.cordic.maximumShiftValue(u));
    else
        N = coder.const(maximumShiftValue);
    end

    Kn = coder.const(fixed.cordic.hyperbolic.inverseScaleFactor(N));
    INITOFFSET = coder.const(0.25);
    shiftSeq = coder.const(fixed.cordic.hyperbolic.shiftSequence(N));
    nCORDICIterations = coder.const(length(shiftSeq));

    %% Run CORDIC square root workflow
    uPos = fixed.cordic.linear.makeRealScalarPositiveUnsigned(u);
    if isfi(u)&&isscaledtype(u)
        coder.internal.assert(u.WordLength>N,'fixed:emblib:CORDICMaxShiftValMustBeSmallerThanWordlength');
        [dataOut, eOut, isZero, validOut] = sqrtIterFixed(uPos, validIn, restart,nIterPerReg,Kn,INITOFFSET,shiftSeq,nCORDICIterations);
    else
        [dataOut, eOut] = fixed.emblib.cordicsqrt.cordicSqrtFloat(uPos, Kn, INITOFFSET, shiftSeq, nCORDICIterations);
        validOut = validIn;
        isZero = u==0;
    end
end

function [dataOut, eOut, isZero, validOut] = sqrtIterFixed(u, validIn, restart, nIterPerReg, Kn, INITOFFSET, shiftSeq, nCORDICIterations)
        uInt = stripscaling(u);
        
        wordLength = coder.const(uInt.WordLength);
        normalizerType = numerictype(1,32,0);

        % CORDIC datatype and corresponding fimath
        CORDICprototype = fi([],1,wordLength,wordLength-2,'DataType',uInt.DataType);
        Fxy = fixed.fimathLike(CORDICprototype);
        
        % Allocate registers
        [numOfNormSteps,nNormReg,normInd,nTrailingNormSteps,trailingNormIdx,nLeadingCORDICSteps,nCORDICReg,CORDICShiftInd,nTotReg]...
            = fixed.emblib.cordicsqrt.allocateReg(wordLength,nCORDICIterations,nIterPerReg);
        
        %% Registers
        persistent xRegNorm xRegCORDIC yReg eRegNorm eRegCORDIC validReg dataOutReg eOutReg isZeroReg
        if isempty(xRegNorm)
            xRegNorm = zeros(nNormReg,1,'like',uInt);
            xRegCORDIC = setfimath(zeros(nCORDICReg,1,'like',CORDICprototype),Fxy);
            yReg = setfimath(zeros(nCORDICReg,1,'like',CORDICprototype),Fxy);
            eRegNorm = fi(zeros(nNormReg,1),0,numOfNormSteps,0);
            eRegCORDIC = fi(zeros(nCORDICReg,1),normalizerType);
            validReg = false(nTotReg+1,1);
            dataOutReg = setfimath(cast(0,'like',CORDICprototype),Fxy);
            eOutReg = fi(0,normalizerType);
            isZeroReg = false(nTotReg+1,1);
        end
        
        %% Assign outputs
        dataOut = dataOutReg;
        eOut = eOutReg;
        validOut = validReg(end);
        isZero = isZeroReg(end);
        
        %% Update registers
        [xRegNorm, xRegCORDIC, yReg, eRegNorm, eRegCORDIC, validReg, dataOutReg, eOutReg, isZeroReg]...
        = fixed.emblib.cordicsqrt.cordicSqrtFiScaledtypeUpdateReg(u, uInt, validIn, restart,... % Inputs
        xRegNorm, xRegCORDIC, yReg, eRegNorm, eRegCORDIC, validReg, dataOutReg, eOutReg, isZeroReg,... %Registers
        Kn, INITOFFSET, shiftSeq, nIterPerReg,... % Constants for algorithms
        nTotReg, nNormReg, CORDICShiftInd, normInd, nTrailingNormSteps, trailingNormIdx, nLeadingCORDICSteps); % Constants for partition algorithms
end

== matlab function gm_hdl_model_fixed_vnl/Subsystem1/Subsystem Reference/Absolute of Complex/CORDIC Square Root HDL Optimized1/Bit Shift Arithmetic/embmathops_c6_s5qJlWhB5AyunXvC1Wsa7cH_Bit_Shift_Arithmetic ==
  settings: fimath=hdlfimath
  data: u input; y output; e input; isZero input
function y = bitShiftArithmetic(u,e,isZero)
%#codegen
if isZero
    y = cast(0,'like',u);
else
    if e<0
        y = bitsll(u,-e);
    else
        y = bitsra(u,e);
    end
end

== matlab function gm_hdl_model_fixed_vnl/Subsystem1/Subsystem Reference/CORDIC Square Root HDL Optimized/Bit Shift Arithmetic/embmathops_c6_sxviEMGenxpVSWTChSq0GHG_Bit_Shift_Arithmetic ==
  settings: fimath=hdlfimath
  data: u input; y output; e input; isZero input
function y = bitShiftArithmetic(u,e,isZero)
%#codegen
if isZero
    y = cast(0,'like',u);
else
    if e<0
        y = bitsll(u,-e);
    else
        y = bitsra(u,e);
    end
end

== matlab function gm_hdl_model_fixed_vnl/Subsystem1/Subsystem Reference/CORDIC Square Root HDL Optimized/Cast to Union of Types/slutils_c1_sUkuwzpcxqKl25e4GzDa0OH_Cast_to_Union_of_Types ==
  settings: fimath=hdlfimath
  data: Xref input; Cout output; Cin input
function Cout = castToUnionType(Xref,Cin)
    %castToUnionType Cast second input to union of the two types
    if (isfloat(Xref) && isfloat(Cin)) || (isFixed(Xref) && isFixed(Cin))
        T = fixed.internal.type.unionPrototype(Cin,Xref,...
        'RoundingMethod','Floor',...
        'OverflowAction','Wrap');
        Cout = cast(Cin,'like',T);
    else
        coder.internal.assert(false,'fixed:emblib:InputOutputMustBeAllFixedOrFloat');
    end
end

function t = isFixed(x)
    t = (isfi(x) || isa(x,'embedded.numerictype')) && isscalingbinarypoint(x) ...
        || isinteger(x);
end

== matlab function gm_hdl_model_fixed_vnl/Subsystem1/Subsystem Reference/Real Divide HDL Optimized/ForEach - Real Divide_instance1/Shift and cast to output type/Cast to Union of Types/slutils_c1_sfkclysknIFh6pVVpTDebQG_Cast_to_Union_of_Types ==
  settings: fimath=hdlfimath
  data: Xref input; Cout output; Cin input
function Cout = castToUnionType(Xref,Cin)
    %castToUnionType Cast second input to union of the two types
    if (isfloat(Xref) && isfloat(Cin)) || (isFixed(Xref) && isFixed(Cin))
        T = fixed.internal.type.unionPrototype(Cin,Xref,...
        'RoundingMethod','Floor',...
        'OverflowAction','Wrap');
        Cout = cast(Cin,'like',T);
    else
        coder.internal.assert(false,'fixed:emblib:InputOutputMustBeAllFixedOrFloat');
    end
end

function t = isFixed(x)
    t = (isfi(x) || isa(x,'embedded.numerictype')) && isscalingbinarypoint(x) ...
        || isinteger(x);
end
